simulink model "SlidingMode_HW2"  (R2021a)
settings: Solver=VariableStepAuto  StartTime=0.0  StopTime=10.0  RelTol=1e-3
settings Model: Creator=kiankhaneghahi  LastModifiedBy=kiankhaneghahi
settings SolverCC: ZeroCrossAlgorithm=Adaptive
settings DebuggingCC: IgnoredZcDiagnostic=none

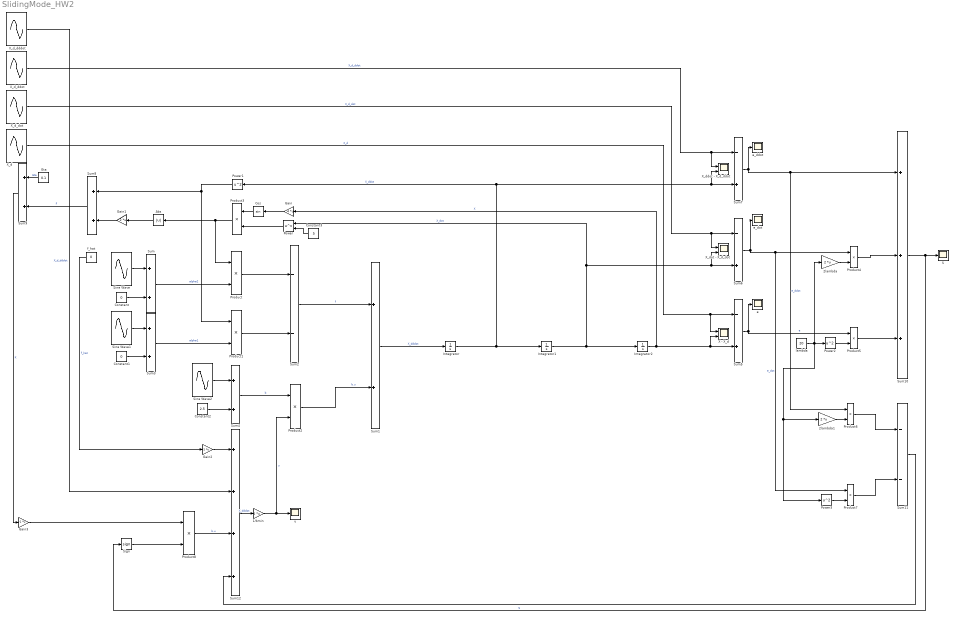
== system SlidingMode_HW2 ==
  1/bmin : Gain  Multiplication=Matrix(K*u)
  2lambda : Gain  Gain=2  Multiplication=Matrix(K*u)
  2lambda1 : Gain  Gain=2  Multiplication=Matrix(K*u)
  Abs : Abs
  Constant : Constant  Value=0
  Constant1 : Constant  Value=0
  Constant2 : Constant  Value=2.5
  Constant3 : Constant  Value=5
  Cos : Trigonometry
  Eta : Constant  Value=0.1
  Gain : Gain  Gain=4  Multiplication=Matrix(K*u)
  Gain1 : Gain  Gain=2  Multiplication=Matrix(K*u)
  Gain2 : Gain  Gain=-1  Multiplication=Matrix(K*u)
  Gain3 : Gain  Gain=-1  Multiplication=Matrix(K*u)
  Integrator : Integrator
  Integrator1 : Integrator
  Integrator2 : Integrator
  Power : Math  Operator=pow  SaturateOnIntegerOverflow=on
  Power1 : Math  Operator=square  SaturateOnIntegerOverflow=on
  Power2 : Math  Operator=square  SaturateOnIntegerOverflow=on
  Power3 : Math  Operator=square  SaturateOnIntegerOverflow=on
  Product{,1..8} (9 alike) : Product
  S : Scope
  Sign : Signum
  Sine Wave : Sin  Amplitude=2  SampleTime=0
  Sine Wave1 : Sin  SampleTime=0
  Sine Wave2 : Sin  Amplitude=1.5  SampleTime=0
  Sum{,1,3..4,8..9} (6 alike) : Sum
  Sum10 : Sum  Inputs=+++
  Sum11 : Sum  Inputs=--
  Sum12 : Sum  Inputs=++++
  Sum2 : Sum  Inputs=--
  Sum5 : Sum  Inputs=-+
  Sum6 : Sum  Inputs=-+
  Sum7 : Sum  Inputs=-+
  X - X_d : Scope  NumInputPorts=2
  X_d : Sin  Frequency=pi/2  SampleTime=0
  X_d_dddot : Sin  Amplitude=-(pi^3)/8  Frequency=pi/2  Phase=pi/2  SampleTime=0
  X_d_ddot : Sin  Amplitude=-(pi^2)/4  Frequency=pi/2  SampleTime=0
  X_d_dot : Sin  Amplitude=pi/2  Frequency=pi/2  Phase=pi/2  SampleTime=0
  X_ddot - X_d_ddot : Scope  NumInputPorts=2
  X_dot - X_d_dot : Scope  NumInputPorts=2
  e : Scope
  e_ddot : Scope
  e_dot : Scope
  f_hat : Constant  Value=0
  lambda : Constant  Value=20
  u : Scope
  wires:
  Sine Wave/1 -> Sum/1
  Sum/1 -> Product/2  "alpha2"
  Product/1 -> Sum2/1
  Constant/1 -> Sum/2
  Sum2/1 -> Sum1/1  "f"
  Constant1/1 -> Sum3/2
  Sine Wave1/1 -> Sum3/1
  Sum3/1 -> Product1/2  "alpha1"
  Product1/1 -> Sum2/2
  Sine Wave2/1 -> Sum4/1
  Constant2/1 -> Sum4/2
  Sum4/1 -> Product2/1  "b"
  Product2/1 -> Sum1/2  "b.u"
  Sum1/1 -> Integrator/1  "X_dddot"
  Gain/1 -> Cos/1
  Cos/1 -> Product3/1
  Product3/1 -> Abs/1, Product/1
  Power1/1 -> Sum8/1, Product1/1
  Power/1 -> Product3/2
  Constant3/1 -> Power/2
  X_d_dddot/1 -> Sum12/2  "X_d_dddot"
  Integrator1/1 -> Sum6/2, X_dot - X_d_dot/2, Power/1, Integrator2/1  "X_dot"
  X_d/1 -> X - X_d/1, Sum5/1  "X_d"
  Integrator2/1 -> X - X_d/2, Sum5/2, Gain/1  "X"
  X_d_dot/1 -> X_dot - X_d_dot/1, Sum6/1  "X_d_dot"
  Integrator/1 -> Sum7/2, X_ddot - X_d_ddot/2, Power1/1, Integrator1/1  "X_ddot"
  X_d_ddot/1 -> X_ddot - X_d_ddot/1, Sum7/1  "X_d_ddot"
  Abs/1 -> Gain1/1
  Gain1/1 -> Sum8/2
  Sum8/1 -> Sum9/2  "F"
  f_hat/1 -> Gain2/1  "f_hat"
  Sum5/1 -> Product5/1, e/1  "e"
  2lambda/1 -> Product4/2
  Power2/1 -> Product5/2
  Eta/1 -> Sum9/1  "Eta"
  Sum9/1 -> Gain3/1  "K"
  Product4/1 -> Sum10/2
  Product5/1 -> Sum10/3
  Sum10/1 -> S/1, Sign/1  "S"
  2lambda1/1 -> Product6/2
  lambda/1 -> 2lambda1/1, Power3/1, Power2/1, 2lambda/1
  Sum6/1 -> e_dot/1, Product7/1, Product4/1  "e_dot"
  Power3/1 -> Product7/2
  Sum7/1 -> Product6/1, Sum10/1, e_ddot/1  "e_ddot"
  Product6/1 -> Sum11/1
  Product7/1 -> Sum11/2
  Sum11/1 -> Sum12/4
  Sum12/1 -> 1/bmin/1  "X_dddot"
  1/bmin/1 -> u/1, Product2/2  "u"
  Gain2/1 -> Sum12/1
  Product8/1 -> Sum12/3  "b.u"
  Gain3/1 -> Product8/1
  Sign/1 -> Product8/2
